simulink library "PTOSim_Lib"  (R2019b)
settings: Solver=ode45  StartTime=0.0  StopTime=10.0  RelTol=1e-3  EnableMultiTasking=on
undefined symbols (not defined in the file): pAeq, pAupper_limit, pBeq, pBupper_limit, ptosim, table
(part 2 of 2)

== system PTOSim_Lib/Motion Conversion/Rotary to Linear Adjustable Rod/Angular to Linear Velocity ==
  angPos : Inport
  angVel : Inport  Port=2
  Add1 : Sum  Inputs=+-
  Add2 : Sum  Inputs=+-
  Add3 : Sum
  Constant1 : Constant  Value=ptosim.crank
  Constant2 : Constant  Value=ptosim.crank
  Constant3 : Constant  Value=ptosim.offset
  Constant7 : Constant  Value=ptosim.crank
  Distance btw flap joint & rod joint along x-axis : Subsystem
  Divide1 : Product  Inputs=*/
  Product1 : Product  Inputs=**
  Product2 : Product  Inputs=***
  Product3 : Product  Inputs=**
  Product4 : Product  Inputs=***
  Product7 : Product  Inputs=**
  Subsystem : Subsystem
  Trigonometric Function1 : Trigonometry  Operator=cos
  Trigonometric Function2 : Trigonometry  Operator=cos
  Trigonometric Function5 : Trigonometry
  linearVel : Outport
  wires:
  Add2/1 -> Product2/1
  Constant2/1 -> Product1/1
  Trigonometric Function1/1 -> Product1/2
  Product1/1 -> Add2/1
  Constant3/1 -> Add2/2
  Trigonometric Function5/1 -> Product7/2
  Product7/1 -> Add1/1, Product2/2
  Constant7/1 -> Product7/1
  angVel/1 -> Product2/3, Product4/1
  Distance btw flap joint & rod joint along x-axis/1(d) -> Add1/2
  Constant1/1 -> Product3/1
  Trigonometric Function2/1 -> Product3/2
  Product3/1 -> Product4/3
  angPos/1 -> Trigonometric Function5/1, Trigonometric Function2/1, Trigonometric Function1/1, Subsystem/1(angPos)
  Add1/1 -> Product4/2
  Subsystem/1(rodLength) -> Divide1/2
  Product2/1 -> Add3/1
  Product4/1 -> Add3/2
  Add3/1 -> Divide1/1
  Divide1/1 -> linearVel/1

== system PTOSim_Lib/Motion Conversion/Rotary to Linear Adjustable Rod/Subsystem ==
  angPos : Inport
  Add2 : Sum  Inputs=+-
  Add5 : Sum
  Add6 : Sum  Inputs=+-
  Constant2 : Constant  Value=ptosim.crank
  Constant3 : Constant  Value=ptosim.offset
  Constant7 : Constant  Value=ptosim.crank
  Distance btw flap joint & rod joint along x-axis : Subsystem
  Math Function1 : Math  Operator=square  SaturateOnIntegerOverflow=on
  Math Function6 : Math  Operator=square  SaturateOnIntegerOverflow=on
  Product1 : Product  Inputs=**
  Product7 : Product  Inputs=**
  Sqrt2 : Sqrt  SaturateOnIntegerOverflow=on
  Trigonometric Function1 : Trigonometry  Operator=cos
  Trigonometric Function5 : Trigonometry
  rodLength : Outport
  wires:
  angPos/1 -> Trigonometric Function5/1, Trigonometric Function1/1
  Add2/1 -> Math Function1/1
  Trigonometric Function5/1 -> Product7/2
  Product7/1 -> Add6/2
  Add6/1 -> Math Function6/1
  Math Function6/1 -> Add5/2
  Add5/1 -> Sqrt2/1
  Sqrt2/1 -> rodLength/1
  Constant2/1 -> Product1/1
  Trigonometric Function1/1 -> Product1/2
  Product1/1 -> Add2/1
  Constant3/1 -> Add2/2
  Math Function1/1 -> Add5/1
  Constant7/1 -> Product7/1
  Distance btw flap joint & rod joint along x-axis/1(d) -> Add6/1

== system PTOSim_Lib/Motion Conversion/Rotary to Linear Crank/Angular to Linear Position ==
  angPos : Inport
  Add1 : Sum  Inputs=++-
  Add2 : Sum  Inputs=+-
  Add5 : Sum  Inputs=+-
  Constant1 : Constant  Value=ptosim.rodLength
  Constant2 : Constant  Value=ptosim.crank
  Constant3 : Constant  Value=ptosim.offset
  Constant7 : Constant  Value=ptosim.crank
  Initial Distance btw flap joint & crank joint along x-axis : Subsystem
  Math Function1 : Math  Operator=square  SaturateOnIntegerOverflow=on
  Math Function2 : Math  Operator=square  SaturateOnIntegerOverflow=on
  Product1 : Product  Inputs=**
  Product7 : Product  Inputs=**
  Sqrt2 : Sqrt  SaturateOnIntegerOverflow=on
  Trigonometric Function1 : Trigonometry  Operator=cos
  Trigonometric Function5 : Trigonometry
  linearPos : Outport
  wires:
  angPos/1 -> Trigonometric Function1/1, Trigonometric Function5/1
  Add2/1 -> Math Function1/1
  Trigonometric Function5/1 -> Product7/2
  Add5/1 -> Sqrt2/1
  Constant2/1 -> Product1/1
  Trigonometric Function1/1 -> Product1/2
  Product1/1 -> Add2/1
  Constant3/1 -> Add2/2
  Constant7/1 -> Product7/1
  Initial Distance btw flap joint & crank joint along x-axis/1(d) -> Add1/3
  Constant1/1 -> Math Function2/1
  Math Function1/1 -> Add5/2
  Sqrt2/1 -> Add1/2
  Product7/1 -> Add1/1
  Add1/1 -> linearPos/1
  Math Function2/1 -> Add5/1

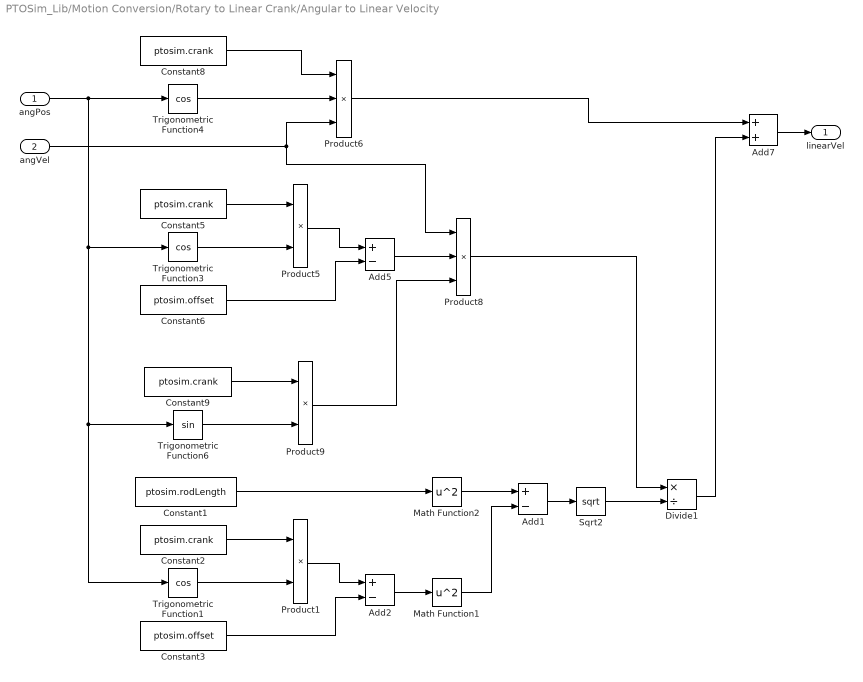
== system PTOSim_Lib/Motion Conversion/Rotary to Linear Crank/Angular to Linear Velocity ==
  angPos : Inport
  angVel : Inport  Port=2
  Add1 : Sum  Inputs=+-
  Add2 : Sum  Inputs=+-
  Add5 : Sum  Inputs=+-
  Add7 : Sum
  Constant1 : Constant  Value=ptosim.rodLength
  Constant{2,5,8..9} (4 alike) : Constant  Value=ptosim.crank
  Constant3 : Constant  Value=ptosim.offset
  Constant6 : Constant  Value=ptosim.offset
  Divide1 : Product  Inputs=*/
  Math Function1 : Math  Operator=square  SaturateOnIntegerOverflow=on
  Math Function2 : Math  Operator=square  SaturateOnIntegerOverflow=on
  Product1 : Product  Inputs=**
  Product5 : Product  Inputs=**
  Product6 : Product  Inputs=***
  Product8 : Product  Inputs=***
  Product9 : Product  Inputs=**
  Sqrt2 : Sqrt  SaturateOnIntegerOverflow=on
  Trigonometric Function1 : Trigonometry  Operator=cos
  Trigonometric Function3 : Trigonometry  Operator=cos
  Trigonometric Function4 : Trigonometry  Operator=cos
  Trigonometric Function6 : Trigonometry
  linearVel : Outport
  wires:
  Add7/1 -> linearVel/1
  Trigonometric Function4/1 -> Product6/2
  Constant8/1 -> Product6/1
  Product6/1 -> Add7/1
  Constant5/1 -> Product5/1
  Trigonometric Function3/1 -> Product5/2
  Product5/1 -> Add5/1
  Constant6/1 -> Add5/2
  Constant9/1 -> Product9/1
  Trigonometric Function6/1 -> Product9/2
  angVel/1 -> Product8/1, Product6/3
  Add5/1 -> Product8/2
  Product9/1 -> Product8/3
  angPos/1 -> Trigonometric Function1/1, Trigonometric Function6/1, Trigonometric Function3/1, Trigonometric Function4/1
  Add2/1 -> Math Function1/1
  Add1/1 -> Sqrt2/1
  Constant2/1 -> Product1/1
  Trigonometric Function1/1 -> Product1/2
  Product1/1 -> Add2/1
  Constant3/1 -> Add2/2
  Constant1/1 -> Math Function2/1
  Math Function1/1 -> Add1/2
  Sqrt2/1 -> Divide1/2
  Product8/1 -> Divide1/1
  Divide1/1 -> Add7/2
  Math Function2/1 -> Add1/1

== system PTOSim_Lib/Motion Conversion/Rotary to Linear Adjustable Rod/Angular to Linear Position/Distance btw flap joint & rod joint along x-axis ==
  Add3 : Sum  Inputs=+-
  Add4 : Sum  Inputs=+-
  Constant4 : Constant  Value=ptosim.rodInit
  Constant5 : Constant  Value=ptosim.crank
  Constant6 : Constant  Value=ptosim.offset
  Math Function2 : Math  Operator=square  SaturateOnIntegerOverflow=on
  Math Function3 : Math  Operator=square  SaturateOnIntegerOverflow=on
  Sqrt1 : Sqrt  SaturateOnIntegerOverflow=on
  d : Outport
  wires:
  Add3/1 -> Sqrt1/1
  Constant4/1 -> Math Function2/1
  Constant5/1 -> Add4/1
  Constant6/1 -> Add4/2
  Add4/1 -> Math Function3/1
  Math Function3/1 -> Add3/2
  Math Function2/1 -> Add3/1
  Sqrt1/1 -> d/1

== system PTOSim_Lib/Motion Conversion/Rotary to Linear Adjustable Rod/Angular to Linear Velocity/Distance btw flap joint & rod joint along x-axis ==
  Add3 : Sum  Inputs=+-
  Add4 : Sum  Inputs=+-
  Constant4 : Constant  Value=ptosim.rodInit
  Constant5 : Constant  Value=ptosim.crank
  Constant6 : Constant  Value=ptosim.offset
  Math Function2 : Math  Operator=square  SaturateOnIntegerOverflow=on
  Math Function3 : Math  Operator=square  SaturateOnIntegerOverflow=on
  Sqrt1 : Sqrt  SaturateOnIntegerOverflow=on
  d : Outport
  wires:
  Add3/1 -> Sqrt1/1
  Constant4/1 -> Math Function2/1
  Constant5/1 -> Add4/1
  Constant6/1 -> Add4/2
  Add4/1 -> Math Function3/1
  Math Function3/1 -> Add3/2
  Math Function2/1 -> Add3/1
  Sqrt1/1 -> d/1

== system PTOSim_Lib/Motion Conversion/Rotary to Linear Adjustable Rod/Angular to Linear Velocity/Subsystem ==
  angPos : Inport
  Add2 : Sum  Inputs=+-
  Add5 : Sum
  Add6 : Sum  Inputs=+-
  Constant2 : Constant  Value=ptosim.crank
  Constant3 : Constant  Value=ptosim.offset
  Constant7 : Constant  Value=ptosim.crank
  Distance btw flap joint & rod joint along x-axis : Subsystem
  Math Function1 : Math  Operator=square  SaturateOnIntegerOverflow=on
  Math Function6 : Math  Operator=square  SaturateOnIntegerOverflow=on
  Product1 : Product  Inputs=**
  Product7 : Product  Inputs=**
  Sqrt2 : Sqrt  SaturateOnIntegerOverflow=on
  Trigonometric Function1 : Trigonometry  Operator=cos
  Trigonometric Function5 : Trigonometry
  rodLength : Outport
  wires:
  angPos/1 -> Trigonometric Function5/1, Trigonometric Function1/1
  Add2/1 -> Math Function1/1
  Trigonometric Function5/1 -> Product7/2
  Product7/1 -> Add6/2
  Add6/1 -> Math Function6/1
  Math Function6/1 -> Add5/2
  Add5/1 -> Sqrt2/1
  Sqrt2/1 -> rodLength/1
  Constant2/1 -> Product1/1
  Trigonometric Function1/1 -> Product1/2
  Product1/1 -> Add2/1
  Constant3/1 -> Add2/2
  Math Function1/1 -> Add5/1
  Constant7/1 -> Product7/1
  Distance btw flap joint & rod joint along x-axis/1(d) -> Add6/1

== system PTOSim_Lib/Motion Conversion/Rotary to Linear Adjustable Rod/Subsystem/Distance btw flap joint & rod joint along x-axis ==
  Add3 : Sum  Inputs=+-
  Add4 : Sum  Inputs=+-
  Constant4 : Constant  Value=ptosim.rodInit
  Constant5 : Constant  Value=ptosim.crank
  Constant6 : Constant  Value=ptosim.offset
  Math Function2 : Math  Operator=square  SaturateOnIntegerOverflow=on
  Math Function3 : Math  Operator=square  SaturateOnIntegerOverflow=on
  Sqrt1 : Sqrt  SaturateOnIntegerOverflow=on
  d : Outport
  wires:
  Add3/1 -> Sqrt1/1
  Constant4/1 -> Math Function2/1
  Constant5/1 -> Add4/1
  Constant6/1 -> Add4/2
  Add4/1 -> Math Function3/1
  Math Function3/1 -> Add3/2
  Math Function2/1 -> Add3/1
  Sqrt1/1 -> d/1

== system PTOSim_Lib/Motion Conversion/Rotary to Linear Crank/Angular to Linear Position/Initial Distance btw flap joint & crank joint along x-axis ==
  Add3 : Sum  Inputs=+-
  Add4 : Sum  Inputs=+-
  Constant1 : Constant  Value=ptosim.rodLength
  Constant5 : Constant  Value=ptosim.crank
  Constant6 : Constant  Value=ptosim.offset
  Math Function2 : Math  Operator=square  SaturateOnIntegerOverflow=on
  Math Function3 : Math  Operator=square  SaturateOnIntegerOverflow=on
  Sqrt1 : Sqrt  SaturateOnIntegerOverflow=on
  d : Outport
  wires:
  Add3/1 -> Sqrt1/1
  Constant1/1 -> Math Function2/1
  Constant5/1 -> Add4/1
  Constant6/1 -> Add4/2
  Add4/1 -> Math Function3/1
  Math Function3/1 -> Add3/2
  Math Function2/1 -> Add3/1
  Sqrt1/1 -> d/1

== system PTOSim_Lib/Motion Conversion/Rotary to Linear Adjustable Rod/Angular to Linear Velocity/Subsystem/Distance btw flap joint & rod joint along x-axis ==
  Add3 : Sum  Inputs=+-
  Add4 : Sum  Inputs=+-
  Constant4 : Constant  Value=ptosim.rodInit
  Constant5 : Constant  Value=ptosim.crank
  Constant6 : Constant  Value=ptosim.offset
  Math Function2 : Math  Operator=square  SaturateOnIntegerOverflow=on
  Math Function3 : Math  Operator=square  SaturateOnIntegerOverflow=on
  Sqrt1 : Sqrt  SaturateOnIntegerOverflow=on
  d : Outport
  wires:
  Add3/1 -> Sqrt1/1
  Constant4/1 -> Math Function2/1
  Constant5/1 -> Add4/1
  Constant6/1 -> Add4/2
  Add4/1 -> Math Function3/1
  Math Function3/1 -> Add3/2
  Math Function2/1 -> Add3/1
  Sqrt1/1 -> d/1
